simulink model "threelink_simulink_analysis"  (R2015a)
settings: Solver=ode45  StartTime=solversettings.t_start  StopTime=solversettings.t_stop  MaxStep=solversettings.t_sample  RelTol=solversettings.rel_tol  AbsTol=solversettings.abs_tol
undefined symbols (not defined in the file or in its folder): solversettings
libraries: robotlib x7, simulink x2

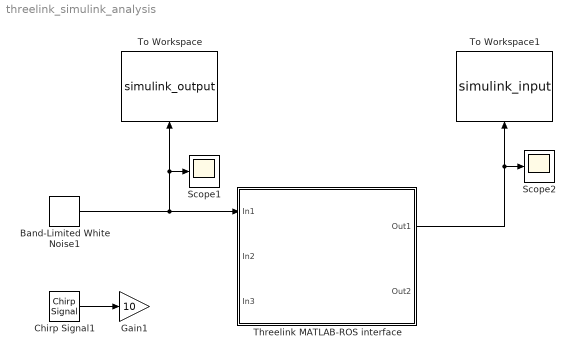
== system threelink_simulink_analysis ==
  Band-Limited White Noise1 : simulink/Sources/Band-Limited White Noise  Cov=[0.01]  Ts=solversettings.t_sample  seed=[round(rand*10000)]
  Chirp Signal1 : simulink/Sources/Chirp Signal  f1=0.01  T=10  f2=100
  Gain1 : Gain  Gain=10
  Scope1 : Scope
  Scope2 : Scope
  Threelink MATLAB-ROS interface : Subsystem
  To Workspace : ToWorkspace  SaveFormat=Timeseries  SampleTime=-1
  To Workspace1 : ToWorkspace  VariableName=simulink_input  SaveFormat=Timeseries  SampleTime=-1
  wires:
  Band-Limited White Noise1/1 -> Scope1/1, To Workspace/1, Threelink MATLAB-ROS interface/1(In1)
  Threelink MATLAB-ROS interface/1(Out1) -> Scope2/1, To Workspace1/1
  Chirp Signal1/1 -> Gain1/1

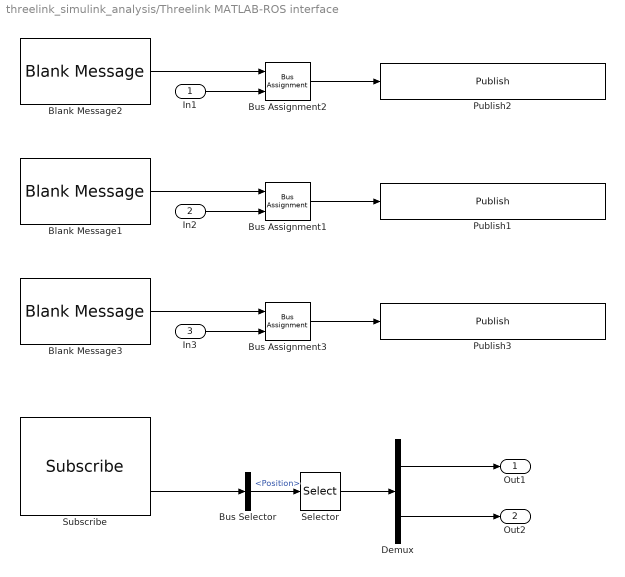
== system threelink_simulink_analysis/Threelink MATLAB-ROS interface ==
  In1 : Inport
  In2 : Inport  Port=2
  In3 : Inport  Port=3
  Blank Message1 : robotlib/Blank Message  SourceLibraryInfo=This block requires Robotics System Toolbox  messageType=std_msgs/Float64  SampleTime=inf
  Blank Message2 : robotlib/Blank Message  SourceLibraryInfo=This block requires Robotics System Toolbox  messageType=std_msgs/Float64  SampleTime=inf
  Blank Message3 : robotlib/Blank Message  SourceLibraryInfo=This block requires Robotics System Toolbox  messageType=std_msgs/Float64  SampleTime=inf
  Bus Assignment1 : BusAssignment  AssignedSignals=Data
  Bus Assignment2 : BusAssignment  AssignedSignals=Data
  Bus Assignment3 : BusAssignment  AssignedSignals=Data
  Bus Selector : BusSelector  OutputSignals=Position
  Demux : Demux  Outputs=2
  Publish1 : robotlib/Publish  SourceLibraryInfo=This block requires Robotics System Toolbox  topicSource=Specify your own  topic=/threelink/joint_2_effort_controller/command  messageType=std_msgs/Float64  messageQueueLength=1
  Publish2 : robotlib/Publish  SourceLibraryInfo=This block requires Robotics System Toolbox  topicSource=Specify your own  topic=/threelink/joint_1_effort_controller/command  messageType=std_msgs/Float64  messageQueueLength=1
  Publish3 : robotlib/Publish  SourceLibraryInfo=This block requires Robotics System Toolbox  topicSource=Specify your own  topic=/threelink/joint_3_effort_controller/command  messageType=std_msgs/Float64  messageQueueLength=1
  Selector : Selector  InputPortWidth=128  Indices=[1 2]
  Subscribe : robotlib/Subscribe  SourceLibraryInfo=This block requires Robotics System Toolbox  topicSource=Specify your own  topic=/threelink/joint_states  messageType=sensor_msgs/JointState  sampleTime=-1  messageQueueLength=1
  Out1 : Outport
  Out2 : Outport  Port=2
  wires:
  Blank Message1/1 -> Bus Assignment1/1
  Bus Assignment1/1 -> Publish1/1
  Blank Message2/1 -> Bus Assignment2/1
  Bus Assignment2/1 -> Publish2/1
  In1/1 -> Bus Assignment2/2
  In2/1 -> Bus Assignment1/2
  Subscribe/2 -> Bus Selector/1
  Bus Selector/1 -> Selector/1  "<Position>"
  Selector/1 -> Demux/1
  Demux/1 -> Out1/1
  Demux/2 -> Out2/1
  Blank Message3/1 -> Bus Assignment3/1
  Bus Assignment3/1 -> Publish3/1
  In3/1 -> Bus Assignment3/2
